simulink model "systemDiagram"  (R2019b)
settings: Solver=VariableStepAuto  StartTime=0.0  StopTime=10.0  RelTol=1e-3
settings Model: Creator=robeshel  LastModifiedBy=robeshel

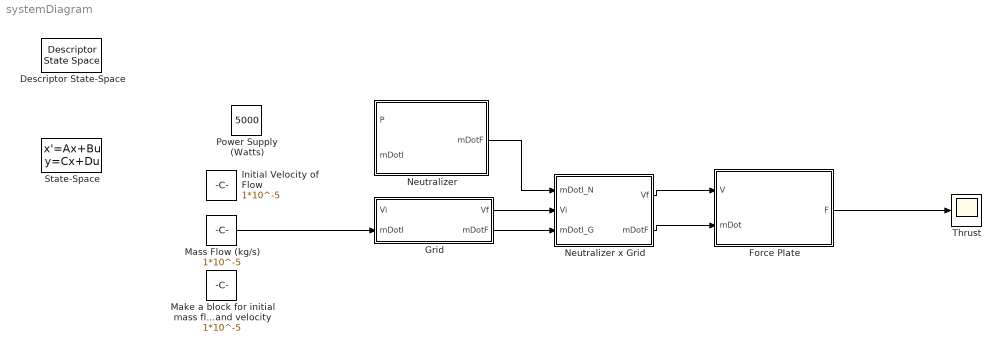
== system systemDiagram ==
  Descriptor State-Space : DescriptorStateSpace
  Force Plate : MATLAB Function  TreatAsAtomicUnit=on
  Grid : MATLAB Function  TreatAsAtomicUnit=on
  Initial Velocity of Flow : Constant  Value=1*10^-5
  Make a block for initial mass flow and velocity : Constant  Value=1*10^-5
  Mass Flow (kg/s) : Constant  Value=1*10^-5
  Neutralizer : MATLAB Function  TreatAsAtomicUnit=on
  Neutralizer x Grid : MATLAB Function  TreatAsAtomicUnit=on
  Power Supply (Watts) : Constant  Value=5000
  State-Space : StateSpace  InitialCondition=0
  Thrust : Scope
  wires:
  Force Plate/1(F) -> Thrust/1
  Neutralizer x Grid/1(Vf) -> Force Plate/1(V)
  Neutralizer x Grid/2(mDotF) -> Force Plate/2(mDot)
  Grid/2(mDotF) -> Neutralizer x Grid/3(mDotI_G)
  Grid/1(Vf) -> Neutralizer x Grid/2(Vi)
  Neutralizer/1(mDotF) -> Neutralizer x Grid/1(mDotI_N)
  Mass Flow (kg/s)/1 -> Grid/2(mDotI)

== matlab function systemDiagram/Grid ==
  data: Vi input; Vf output; mDotI input; mDotF output
function [Vf,mDotF]= fcn(Vi,mDotI)

mDotF = mDotI - 123;
Vf = Vi / 2;

== matlab function systemDiagram/Neutralizer x Grid ==
  data: mDotI_N input; Vf output; mDotF output; Vi input; mDotI_G input
function [Vf,mDotF]= fcn(mDotI_N, Vi, mDotI_G)

Vf = Vi * 0.5;
if(mDotI_N > 100)
    mDotF = mDotI_G / 2;
end

== matlab function systemDiagram/Force Plate ==
  data: V input; F output; mDot input
function F = fcn(V, mDot)

%thrust equation of an ion engine
F = V * mDot;

== matlab function systemDiagram/Neutralizer ==
  data: P input; mDotI input; mDotF output
function mDotF = fcn(P,mDotI)

mDotF = mDotI * P;
